simulink model "weixing3_pd_ekf1"  (R2019a)
settings: Solver=FixedStepAuto  StartTime=0.0  StopTime=40  FixedStep=0.001  RelTol=1e-3  EnableMultiTasking=on
values from neighbouring files (symbols this model uses):
  f = Jn\M(:,i)    [Copy_of_flexcont_Slidemode.m]    (also in flash.m = getframe(gcf); flexcont1_wb.m = -H'*wv(:,i); flexcont2.m; flexcont2_wb.m)
libraries: instrumentlib x2, simulink x1
settings Model: Creator=Administrator  LastModifiedBy=HP
settings DataIOCC: ExternalInput=[t, y]  LimitDataPoints=on  MaxDataPoints=15000  ReturnWorkspaceOutputs=off
settings OptimizationCC: LifeSpan=inf
settings DebuggingCC: MultiTaskCondExecSysMsg=warning  MultiTaskRateTransMsg=warning  AllowSymbolicDim=off  SFUnexpectedBacktrackingDiag=warning  SFNoUnconditionalDefaultTransitionDiag=warning  SFExecutionAtInitializationDiag=none  ArithmeticOperatorsInVariantConditions=warning
settings ModelReferenceCC: PropagateSignalLabelsOutOfModel=off
settings SFSimCC: SimUseLocalCustomCode=off
settings RTWCC: RTWUseLocalCustomCode=off
settings CodeAppCC: StateflowObjectComments=on
settings GRTTargetCC: TargetLangStandard=C89/C90 (ANSI)
settings ConfigComp: CovMetricSettings=dw  CovHtmlReporting=on  CovSaveCumulativeToWorkspaceVar=on  CovSaveSingleToWorkspaceVar=on  CovExternalEMLEnable=off

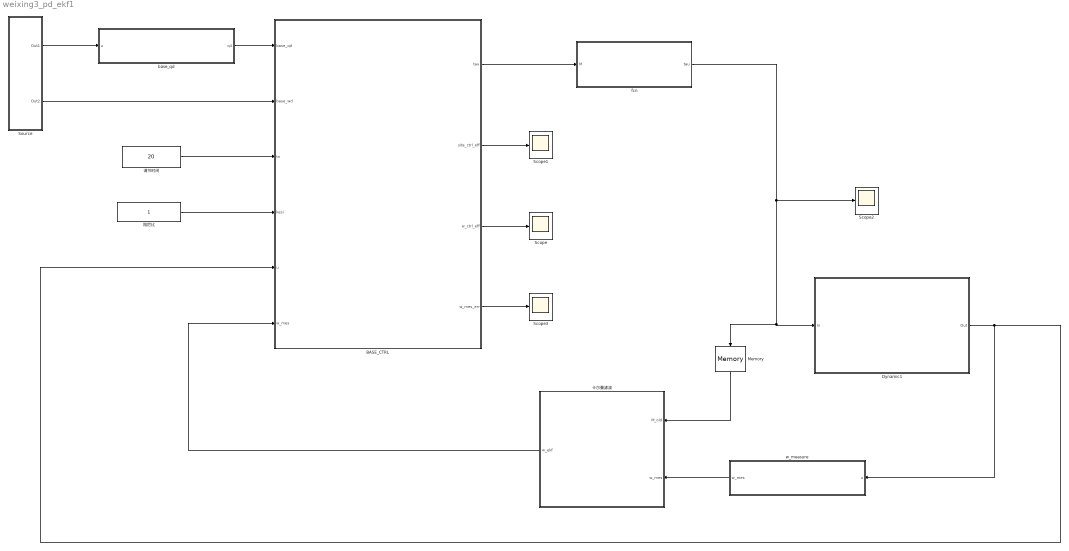
== system weixing3_pd_ekf1 ==
  " Dynamic1" : Subsystem  Description=|  mask{com_step=0.001, tcp_data_size=16, host_name=localhost, tcp_port=50028, tcp_timeout=15}
      | This block can be used to exchange data with Chrono::Engine.                                                                                      
      | A Chrono::Engine program with a running ChCosimulation inferface must be started, it will work as a server; then the Simulink program must be run.
      | Note! check that the dimensions of the exchanged vectors do match!
      mask prompts: com_step "Communication step size"; tcp_data_size "N. of scalars received from C::E (as block output)"; host_name "TCP host name (ex. 'localhost', or 'www.myhost.com')"; tcp_port "TCP port (ex. 50007)"; tcp_timeout "TCP timeout (seconds)"
      mask init:
      | block_receive = [gcb, '/TCP Receive'];
      | set_param(block_receive, 'SampleTime', num2str(com_step));
      | set_param(block_receive, 'Host', host_name);
      | set_param(block_receive, 'Port', num2str(tcp_port));
      | set_param(block_receive, 'DataSize', num2str(tcp_data_size));
      | set_param(block_receive, 'Timeout', num2str(tcp_timeout));
      | block_send = [gcb, '/TCP Send'];
      | set_param(block_send, 'Host', host_name);
      | set_param(block_send, 'Port', num2str(tcp_port));
      mask Display: disp('MBSim CoSim/Matlab')
  BASE_CTRL : MATLAB Function  TreatAsAtomicUnit=on
  Memory : Memory  InitialCondition=[zeros(9,1);1]
  Scope{,1..3} (4 alike) : Scope
  Source : Subsystem
  base_qd : MATLAB Function  TreatAsAtomicUnit=on
  fcn : MATLAB Function  TreatAsAtomicUnit=on
  w_measure : MATLAB Function  TreatAsAtomicUnit=on
  卡尔曼滤波 : MATLAB Function  TreatAsAtomicUnit=on
  调节时间 : Constant  Value=20
  阻尼比 : Constant
  wires:
  base_qd/1(q4) -> BASE_CTRL/1(base_qd)
  Source/2(Out2) -> BASE_CTRL/2(base_wd)
  调节时间/1 -> BASE_CTRL/3(tn)
  阻尼比/1 -> BASE_CTRL/4(kesi)
  BASE_CTRL/3(w_ctrl_eff) -> Scope/1
  BASE_CTRL/2(sita_ctrl_eff) -> Scope1/1
  " Dynamic1"/1(Out) -> w_measure/1(u), BASE_CTRL/5(u)
  Source/1(Out1) -> base_qd/1(u)
  BASE_CTRL/1(tau) -> fcn/1(M)
  fcn/1(tau) -> Scope2/1, Memory/1, " Dynamic1"/1(In)
  BASE_CTRL/4(w_mes_err) -> Scope3/1
  w_measure/1(w_mes) -> 卡尔曼滤波/2(w_mes)
  卡尔曼滤波/1(w_ekf) -> BASE_CTRL/6(w_mes)
  Memory/1 -> 卡尔曼滤波/1(M_old)

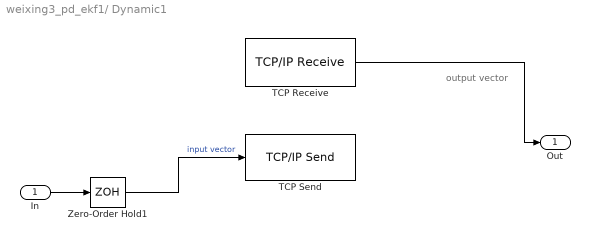
== system weixing3_pd_ekf1/ Dynamic1 ==
  note: output vector
  In : Inport
  TCP Receive : instrumentlib/TCP//IP Receive  Priority=1  Host=localhost  Port=50028  DataSize=16  EnableBlockingMode=on  Timeout=15  SampleTime=0.001  DataType=double  ByteOrder=LittleEndian  ASCIIFormatting=%f,  Terminator=LF
      settings: SourceProductName=Instrument Control Toolbox
  TCP Send : instrumentlib/TCP//IP Send  Priority=2  Host=localhost  Port=50028  EnableBlockingMode=off  Timeout=10  ByteOrder=LittleEndian  TransferDelay=on
      settings: SourceProductName=Instrument Control Toolbox
  Zero-Order Hold1 : ZeroOrderHold  SampleTime=com_step
  Out : Outport
  wires:
  Zero-Order Hold1/1 -> TCP Send/1  "input vector"
  In/1 -> Zero-Order Hold1/1
  TCP Receive/1 -> Out/1

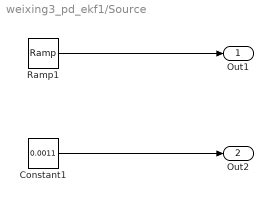
== system weixing3_pd_ekf1/Source ==
  Constant1 : Constant  Value=0.0011
  Ramp1 : simulink/Sources/Ramp  slope=0.0011  start=0  InitialOutput=0
  Out1 : Outport
  Out2 : Outport  Port=2
  wires:
  Constant1/1 -> Out2/1
  Ramp1/1 -> Out1/1

== matlab function weixing3_pd_ekf1/base_qd ==
  data: u input; q4 output
function q4 = fcn(u)
    base_qd=zeros(4,1);
    base_qd(1)=cos(u/2);
    base_qd(2)=sin(u/2);
    q1=[cos(-10*pi/180/2);0;sin(-10*pi/180/2);0];
    q2=[cos(-10*pi/180/2);sin(-10*pi/180/2);0;0];
    q3=[q1(1) -q1(2) -q1(3) -q1(4);
    q1(2) q1(1) -q1(4) q1(3);
    q1(3) q1(4) q1(1) -q1(2);
    q1(4) -q1(3) q1(2) q1(1)]*q2;
    q4=[q3(1) -q3(2) -q3(3) -q3(4);
    q3(2) q3(1) -q3(4) q3(3);
    q3(3) q3(4) q3(1) -q3(2);
    q3(4) -q3(3) q3(2) q3(1)]*base_qd;
end

== matlab function weixing3_pd_ekf1/w_measure ==
  data: u input; w_mes output
function w_mes = fcn(u)
base_q=u(6:9);
base_qv=u(13:16);
w=2*[-base_q(2),base_q(1),base_q(4),-base_q(3);
    -base_q(3),-base_q(4),base_q(1),base_q(2);
    -base_q(4),base_q(3),-base_q(2),base_q(1)]*base_qv;
noise_mes=8e-04;%1sigm  0.1deg/s(3sigm)
w_mes=w+noise_mes*randn(3,1);
end

== matlab function weixing3_pd_ekf1/BASE_CTRL ==
  data: tau output; sita_ctrl_eff output; w_ctrl_eff output; base_qd input; base_wd input; tn input; kesi input; u input; w_mes input; w_mes_err output
function [tau,sita_ctrl_eff,w_ctrl_eff,w_mes_err]  =fcn(base_qd,base_wd,tn,kesi,u,w_mes)
%%%%%MBSim输出信息
time=u(1);
time_step=u(2);
base_p=u(3:5);
base_q=u(6:9);
base_pv=u(10:12);
base_qv=u(13:16);

% %测量星体角速度（在本体系下）/滤波得到
w=w_mes;

%构造角速度叉乘矩阵
W=[0 -w(3) w(2);w(3) 0 -w(1);-w(2) w(1) 0];
%四元数误差
qe=[base_qd(1),base_qd(2),base_qd(3),base_qd(4);
    -base_qd(2),base_qd(1),base_qd(4),-base_qd(3);
    -base_qd(3),-base_qd(4),base_qd(1),base_qd(2);
    -base_qd(4),base_qd(3),-base_qd(2),base_qd(1)]*base_q;
%取矢量部分
qe1=qe(2:4);
%期望的姿态变换矩阵
A_OBd=[1-2*base_qd(3)^2-2*base_qd(4)^2,2*(base_qd(2)*base_qd(3)-base_qd(1)*base_qd(4)),2*(base_qd(2)*base_qd(4)+base_qd(1)*base_qd(3));
    2*(base_qd(2)*base_qd(3)+base_qd(1)*base_qd(4)),1-2*base_qd(2)^2-2*base_qd(4)^2,2*(base_qd(4)*base_qd(3)-base_qd(1)*base_qd(2));
    2*(base_qd(2)*base_qd(4)-base_qd(1)*base_qd(3)),2*(base_qd(4)*base_qd(3)+base_qd(1)*base_qd(2)),1-2*base_qd(2)^2-2*base_qd(3)^2];
%实际的基体姿态变换矩阵(相对于惯性坐标系)
A_OB=[1-2*base_q(3)^2-2*base_q(4)^2,2*(base_q(2)*base_q(3)-base_q(1)*base_q(4)),2*(base_q(2)*base_q(4)+base_q(1)*base_q(3));
    2*(base_q(2)*base_q(3)+base_q(1)*base_q(4)),1-2*base_q(2)^2-2*base_q(4)^2,2*(base_q(4)*base_q(3)-base_q(1)*base_q(2));
    2*(base_q(2)*base_q(4)-base_q(1)*base_q(3)),2*(base_q(4)*base_q(3)+base_q(1)*base_q(2)),1-2*base_q(2)^2-2*base_q(3)^2];
A_dB=A_OBd\A_OB;%(由误差四元数构成的姿态变换矩阵)
%角速率误差
we=w-[base_wd;0;0];

% %计算固有频率
wn=10/(kesi*tn);
%%%%%%%%%%%%%%控制率设计
%参数选取与计算
k=wn^2*2;
d=2*kesi*wn;
Jn=[566.7165 -3.77077 -3.77077;-3.77077 3658.9667 -3.77077;-3.77077 -3.77077 3705.628];
D=d*Jn;
K4=k*Jn;
%控制率
tau=zeros(3,1);
tau(1:3)=W*Jn*w-K4*qe1-D*we;

%输出指标-欧拉角误差
%根据本体和期望之间的姿态变换矩阵求解欧拉角
sita_ze=atan(-A_dB(1,2)/A_dB(1,1));
sita_ye=asin(A_dB(1,3));
sita_xe=-asin(A_dB(2,3)/cos(sita_ye));
%输出角度单位
sita_ctrl_eff=[sita_xe;sita_ye;sita_ze]*180/pi;
%输出指标-角速度
w_actual=2*[-base_q(2),base_q(1),base_q(4),-base_q(3);
    -base_q(3),-base_q(4),base_q(1),base_q(2);
    -base_q(4),base_q(3),-base_q(2),base_q(1)]*base_qv;
w_ctrl_eff=[w_actual;[base_wd;0;0]]*180/pi;
%输出指标-测量误差
w_mes_err=(w-w_actual)*180/pi;

end

== matlab function weixing3_pd_ekf1/卡尔曼滤波 ==
  data: M_old input; w_mes input; w_ekf output
function w_ekf  = fcn(M_old,w_mes)
%参数设置
noise_mes=8e-04;%1sigm
T=0.001;
%初值
persistent X;
if isempty(X)
    X=[0;0;0];
end 
persistent P;
if isempty(P)
    P=100*eye(3);
end 
%程序主体
w_old=X;
% Q=diag([1e-9,1e-9,1e-9])/1e3;
R=diag([(noise_mes)^2;(noise_mes)^2;(noise_mes)^2]);
Jn=[566.7165 -3.77077 -3.77077;-3.77077 3658.9667 -3.77077;-3.77077 -3.77077 3705.628];
JJ=inv(Jn);
W_old=[0 -w_old(3) w_old(2);w_old(3) 0 -w_old(1);-w_old(2) w_old(1) 0];
%一步预测
X=w_old-T*JJ*W_old*Jn*w_old+T*JJ*M_old(1:3);
%对非线性函数进行一阶泰勒展开
Ix=Jn(1,1);Iy=Jn(2,2);Iz=Jn(3,3);
Ixy=-Jn(1,2);Ixz=-Jn(1,3);Iyz=-Jn(2,3);
wox=w_old(1);
woy=w_old(2);
woz=w_old(3);
F=[ woy*((Iy*T*(Ixz*Iy + Ixy*Iyz))/(Iz*Ixy^2 + 2*Ixy*Ixz*Iyz + Iy*Ixz^2 + Ix*Iyz^2 - Ix*Iy*Iz) + (Iyz*T*(Ixz*Iyz + Ixy*Iz))/(Iz*Ixy^2 + 2*Ixy*Ixz*Iyz + Iy*Ixz^2 + Ix*Iyz^2 - Ix*Iy*Iz)) - wox*((Ixy*T*(Ixz*Iy + Ixy*Iyz))/(Iz*Ixy^2 + 2*Ixy*Ixz*Iyz + Iy*Ixz^2 + Ix*Iyz^2 - Ix*Iy*Iz) - (Ixz*T*(Ixz*Iyz + Ixy*Iz))/(Iz*Ixy^2 + 2*Ixy*Ixz*Iyz + Iy*Ixz^2 + Ix*Iyz^2 - Ix*Iy*Iz)) - woz*((Iyz*T*(Ixz*Iy + Ixy*Iyz))/(Iz*Ixy^2 + 2*Ixy*Ixz*Iyz + Iy*Ixz^2 + Ix*Iyz^2 - Ix*Iy*Iz) + (Iz*T*(Ixz*Iyz + Ixy*Iz))/(Iz*Ixy^2 + 2*Ixy*Ixz*Iyz + Iy*Ixz^2 + Ix*Iyz^2 - Ix*Iy*Iz)) - Ix*((T*woy*(Ixz*Iy + Ixy*Iyz))/(Iz*Ixy^2 + 2*Ixy*Ixz*Iyz + Iy*Ixz^2 + Ix*Iyz^2 - Ix*Iy*Iz) - (T*woz*(Ixz*Iyz + Ixy*Iz))/(Iz*Ixy^2 + 2*Ixy*Ixz*Iyz + Iy*Ixz^2 + Ix*Iyz^2 - Ix*Iy*Iz)) - Ixy*((T*woz*(Iyz^2 - Iy*Iz))/(Iz*Ixy^2 + 2*Ixy*Ixz*Iyz + Iy*Ixz^2 + Ix*Iyz^2 - Ix*Iy*Iz) + (T*wox*(Ixz*Iy + Ixy*Iyz))/(Iz*Ixy^2 + 2*Ixy*Ixz*Iyz + Iy*Ixz^2 + Ix*Iyz^2 - Ix*Iy*Iz)) + Ixz*((T*woy*(Iyz^2 - Iy*Iz))/(Iz*Ixy^2 + 2*Ixy*Ixz*Iyz + Iy*Ixz^2 + Ix*Iyz^2 - Ix*Iy*Iz) + (T*wox*(Ixz*Iyz + Ixy*Iz))/(Iz*Ixy^2 + 2*Ixy*Ixz*Iyz + Iy*Ixz^2 + Ix*Iyz^2 - Ix*Iy*Iz)) + 1,              Ixy*((T*woy*(Ixz*Iy + Ixy*Iyz))/(Iz*Ixy^2 + 2*Ixy*Ixz*Iyz + Iy*Ixz^2 + Ix*Iyz^2 - Ix*Iy*Iz) - (T*woz*(Ixz*Iyz + Ixy*Iz))/(Iz*Ixy^2 + 2*Ixy*Ixz*Iyz + Iy*Ixz^2 + Ix*Iyz^2 - Ix*Iy*Iz)) + wox*((Ixz*T*(Iyz^2 - Iy*Iz))/(Iz*Ixy^2 + 2*Ixy*Ixz*Iyz + Iy*Ixz^2 + Ix*Iyz^2 - Ix*Iy*Iz) - (Ix*T*(Ixz*Iy + Ixy*Iyz))/(Iz*Ixy^2 + 2*Ixy*Ixz*Iyz + Iy*Ixz^2 + Ix*Iyz^2 - Ix*Iy*Iz)) + woy*((Iyz*T*(Iyz^2 - Iy*Iz))/(Iz*Ixy^2 + 2*Ixy*Ixz*Iyz + Iy*Ixz^2 + Ix*Iyz^2 - Ix*Iy*Iz) + (Ixy*T*(Ixz*Iy + Ixy*Iyz))/(Iz*Ixy^2 + 2*Ixy*Ixz*Iyz + Iy*Ixz^2 + Ix*Iyz^2 - Ix*Iy*Iz)) - woz*((Iz*T*(Iyz^2 - Iy*Iz))/(Iz*Ixy^2 + 2*Ixy*Ixz*Iyz + Iy*Ixz^2 + Ix*Iyz^2 - Ix*Iy*Iz) - (Ixz*T*(Ixz*Iy + Ixy*Iyz))/(Iz*Ixy^2 + 2*Ixy*Ixz*Iyz + Iy*Ixz^2 + Ix*Iyz^2 - Ix*Iy*Iz)) + Iy*((T*woz*(Iyz^2 - Iy*Iz))/(Iz*Ixy^2 + 2*Ixy*Ixz*Iyz + Iy*Ixz^2 + Ix*Iyz^2 - Ix*Iy*Iz) + (T*wox*(Ixz*Iy + Ixy*Iyz))/(Iz*Ixy^2 + 2*Ixy*Ixz*Iyz + Iy*Ixz^2 + Ix*Iyz^2 - Ix*Iy*Iz)) + Iyz*((T*woy*(Iyz^2 - Iy*Iz))/(Iz*Ixy^2 + 2*Ixy*Ixz*Iyz + Iy*Ixz^2 + Ix*Iyz^2 - Ix*Iy*Iz) + (T*wox*(Ixz*Iyz + Ixy*Iz))/(Iz*Ixy^2 + 2*Ixy*Ixz*Iyz + Iy*Ixz^2 + Ix*Iyz^2 - Ix*Iy*Iz)),              Ixz*((T*woy*(Ixz*Iy + Ixy*Iyz))/(Iz*Ixy^2 + 2*Ixy*Ixz*Iyz + Iy*Ixz^2 + Ix*Iyz^2 - Ix*Iy*Iz) - (T*woz*(Ixz*Iyz + Ixy*Iz))/(Iz*Ixy^2 + 2*Ixy*Ixz*Iyz + Iy*Ixz^2 + Ix*Iyz^2 - Ix*Iy*Iz)) - wox*((Ixy*T*(Iyz^2 - Iy*Iz))/(Iz*Ixy^2 + 2*Ixy*Ixz*Iyz + Iy*Ixz^2 + Ix*Iyz^2 - Ix*Iy*Iz) - (Ix*T*(Ixz*Iyz + Ixy*Iz))/(Iz*Ixy^2 + 2*Ixy*Ixz*Iyz + Iy*Ixz^2 + Ix*Iyz^2 - Ix*Iy*Iz)) + woy*((Iy*T*(Iyz^2 - Iy*Iz))/(Iz*Ixy^2 + 2*Ixy*Ixz*Iyz + Iy*Ixz^2 + Ix*Iyz^2 - Ix*Iy*Iz) - (Ixy*T*(Ixz*Iyz + Ixy*Iz))/(Iz*Ixy^2 + 2*Ixy*Ixz*Iyz + Iy*Ixz^2 + Ix*Iyz^2 - Ix*Iy*Iz)) - woz*((Iyz*T*(Iyz^2 - Iy*Iz))/(Iz*Ixy^2 + 2*Ixy*Ixz*Iyz + Iy*Ixz^2 + Ix*Iyz^2 - Ix*Iy*Iz) + (Ixz*T*(Ixz*Iyz + Ixy*Iz))/(Iz*Ixy^2 + 2*Ixy*Ixz*Iyz + Iy*Ixz^2 + Ix*Iyz^2 - Ix*Iy*Iz)) - Iyz*((T*woz*(Iyz^2 - Iy*Iz))/(Iz*Ixy^2 + 2*Ixy*Ixz*Iyz + Iy*Ixz^2 + Ix*Iyz^2 - Ix*Iy*Iz) + (T*wox*(Ixz*Iy + Ixy*Iyz))/(Iz*Ixy^2 + 2*Ixy*Ixz*Iyz + Iy*Ixz^2 + Ix*Iyz^2 - Ix*Iy*Iz)) - Iz*((T*woy*(Iyz^2 - Iy*Iz))/(Iz*Ixy^2 + 2*Ixy*Ixz*Iyz + Iy*Ixz^2 + Ix*Iyz^2 - Ix*Iy*Iz) + (T*wox*(Ixz*Iyz + Ixy*Iz))/(Iz*Ixy^2 + 2*Ixy*Ixz*Iyz + Iy*Ixz^2 + Ix*Iyz^2 - Ix*Iy*Iz));
              woz*((Iz*T*(Ixz^2 - Ix*Iz))/(Iz*Ixy^2 + 2*Ixy*Ixz*Iyz + Iy*Ixz^2 + Ix*Iyz^2 - Ix*Iy*Iz) - (Iyz*T*(Ixy*Ixz + Ix*Iyz))/(Iz*Ixy^2 + 2*Ixy*Ixz*Iyz + Iy*Ixz^2 + Ix*Iyz^2 - Ix*Iy*Iz)) - wox*((Ixz*T*(Ixz^2 - Ix*Iz))/(Iz*Ixy^2 + 2*Ixy*Ixz*Iyz + Iy*Ixz^2 + Ix*Iyz^2 - Ix*Iy*Iz) + (Ixy*T*(Ixy*Ixz + Ix*Iyz))/(Iz*Ixy^2 + 2*Ixy*Ixz*Iyz + Iy*Ixz^2 + Ix*Iyz^2 - Ix*Iy*Iz)) - woy*((Iyz*T*(Ixz^2 - Ix*Iz))/(Iz*Ixy^2 + 2*Ixy*Ixz*Iyz + Iy*Ixz^2 + Ix*Iyz^2 - Ix*Iy*Iz) - (Iy*T*(Ixy*Ixz + Ix*Iyz))/(Iz*Ixy^2 + 2*Ixy*Ixz*Iyz + Iy*Ixz^2 + Ix*Iyz^2 - Ix*Iy*Iz)) - Ixy*((T*wox*(Ixy*Ixz + Ix*Iyz))/(Iz*Ixy^2 + 2*Ixy*Ixz*Iyz + Iy*Ixz^2 + Ix*Iyz^2 - Ix*Iy*Iz) - (T*woz*(Ixz*Iyz + Ixy*Iz))/(Iz*Ixy^2 + 2*Ixy*Ixz*Iyz + Iy*Ixz^2 + Ix*Iyz^2 - Ix*Iy*Iz)) - Ix*((T*woz*(Ixz^2 - Ix*Iz))/(Iz*Ixy^2 + 2*Ixy*Ixz*Iyz + Iy*Ixz^2 + Ix*Iyz^2 - Ix*Iy*Iz) + (T*woy*(Ixy*Ixz + Ix*Iyz))/(Iz*Ixy^2 + 2*Ixy*Ixz*Iyz + Iy*Ixz^2 + Ix*Iyz^2 - Ix*Iy*Iz)) - Ixz*((T*wox*(Ixz^2 - Ix*Iz))/(Iz*Ixy^2 + 2*Ixy*Ixz*Iyz + Iy*Ixz^2 + Ix*Iyz^2 - Ix*Iy*Iz) + (T*woy*(Ixz*Iyz + Ixy*Iz))/(Iz*Ixy^2 + 2*Ixy*Ixz*Iyz + Iy*Ixz^2 + Ix*Iyz^2 - Ix*Iy*Iz)), woy*((Ixy*T*(Ixy*Ixz + Ix*Iyz))/(Iz*Ixy^2 + 2*Ixy*Ixz*Iyz + Iy*Ixz^2 + Ix*Iyz^2 - Ix*Iy*Iz) - (Iyz*T*(Ixz*Iyz + Ixy*Iz))/(Iz*Ixy^2 + 2*Ixy*Ixz*Iyz + Iy*Ixz^2 + Ix*Iyz^2 - Ix*Iy*Iz)) - wox*((Ix*T*(Ixy*Ixz + Ix*Iyz))/(Iz*Ixy^2 + 2*Ixy*Ixz*Iyz + Iy*Ixz^2 + Ix*Iyz^2 - Ix*Iy*Iz) + (Ixz*T*(Ixz*Iyz + Ixy*Iz))/(Iz*Ixy^2 + 2*Ixy*Ixz*Iyz + Iy*Ixz^2 + Ix*Iyz^2 - Ix*Iy*Iz)) + woz*((Ixz*T*(Ixy*Ixz + Ix*Iyz))/(Iz*Ixy^2 + 2*Ixy*Ixz*Iyz + Iy*Ixz^2 + Ix*Iyz^2 - Ix*Iy*Iz) + (Iz*T*(Ixz*Iyz + Ixy*Iz))/(Iz*Ixy^2 + 2*Ixy*Ixz*Iyz + Iy*Ixz^2 + Ix*Iyz^2 - Ix*Iy*Iz)) + Iy*((T*wox*(Ixy*Ixz + Ix*Iyz))/(Iz*Ixy^2 + 2*Ixy*Ixz*Iyz + Iy*Ixz^2 + Ix*Iyz^2 - Ix*Iy*Iz) - (T*woz*(Ixz*Iyz + Ixy*Iz))/(Iz*Ixy^2 + 2*Ixy*Ixz*Iyz + Iy*Ixz^2 + Ix*Iyz^2 - Ix*Iy*Iz)) + Ixy*((T*woz*(Ixz^2 - Ix*Iz))/(Iz*Ixy^2 + 2*Ixy*Ixz*Iyz + Iy*Ixz^2 + Ix*Iyz^2 - Ix*Iy*Iz) + (T*woy*(Ixy*Ixz + Ix*Iyz))/(Iz*Ixy^2 + 2*Ixy*Ixz*Iyz + Iy*Ixz^2 + Ix*Iyz^2 - Ix*Iy*Iz)) - Iyz*((T*wox*(Ixz^2 - Ix*Iz))/(Iz*Ixy^2 + 2*Ixy*Ixz*Iyz + Iy*Ixz^2 + Ix*Iyz^2 - Ix*Iy*Iz) + (T*woy*(Ixz*Iyz + Ixy*Iz))/(Iz*Ixy^2 + 2*Ixy*Ixz*Iyz + Iy*Ixz^2 + Ix*Iyz^2 - Ix*Iy*Iz)) + 1,              woy*((Ixy*T*(Ixz^2 - Ix*Iz))/(Iz*Ixy^2 + 2*Ixy*Ixz*Iyz + Iy*Ixz^2 + Ix*Iyz^2 - Ix*Iy*Iz) - (Iy*T*(Ixz*Iyz + Ixy*Iz))/(Iz*Ixy^2 + 2*Ixy*Ixz*Iyz + Iy*Ixz^2 + Ix*Iyz^2 - Ix*Iy*Iz)) - wox*((Ix*T*(Ixz^2 - Ix*Iz))/(Iz*Ixy^2 + 2*Ixy*Ixz*Iyz + Iy*Ixz^2 + Ix*Iyz^2 - Ix*Iy*Iz) - (Ixy*T*(Ixz*Iyz + Ixy*Iz))/(Iz*Ixy^2 + 2*Ixy*Ixz*Iyz + Iy*Ixz^2 + Ix*Iyz^2 - Ix*Iy*Iz)) - Iyz*((T*wox*(Ixy*Ixz + Ix*Iyz))/(Iz*Ixy^2 + 2*Ixy*Ixz*Iyz + Iy*Ixz^2 + Ix*Iyz^2 - Ix*Iy*Iz) - (T*woz*(Ixz*Iyz + Ixy*Iz))/(Iz*Ixy^2 + 2*Ixy*Ixz*Iyz + Iy*Ixz^2 + Ix*Iyz^2 - Ix*Iy*Iz)) + woz*((Ixz*T*(Ixz^2 - Ix*Iz))/(Iz*Ixy^2 + 2*Ixy*Ixz*Iyz + Iy*Ixz^2 + Ix*Iyz^2 - Ix*Iy*Iz) + (Iyz*T*(Ixz*Iyz + Ixy*Iz))/(Iz*Ixy^2 + 2*Ixy*Ixz*Iyz + Iy*Ixz^2 + Ix*Iyz^2 - Ix*Iy*Iz)) + Ixz*((T*woz*(Ixz^2 - Ix*Iz))/(Iz*Ixy^2 + 2*Ixy*Ixz*Iyz + Iy*Ixz^2 + Ix*Iyz^2 - Ix*Iy*Iz) + (T*woy*(Ixy*Ixz + Ix*Iyz))/(Iz*Ixy^2 + 2*Ixy*Ixz*Iyz + Iy*Ixz^2 + Ix*Iyz^2 - Ix*Iy*Iz)) + Iz*((T*wox*(Ixz^2 - Ix*Iz))/(Iz*Ixy^2 + 2*Ixy*Ixz*Iyz + Iy*Ixz^2 + Ix*Iyz^2 - Ix*Iy*Iz) + (T*woy*(Ixz*Iyz + Ixy*Iz))/(Iz*Ixy^2 + 2*Ixy*Ixz*Iyz + Iy*Ixz^2 + Ix*Iyz^2 - Ix*Iy*Iz));
             Ixz*((T*wox*(Ixy*Ixz + Ix*Iyz))/(Iz*Ixy^2 + 2*Ixy*Ixz*Iyz + Iy*Ixz^2 + Ix*Iyz^2 - Ix*Iy*Iz) - (T*woy*(Ixz*Iy + Ixy*Iyz))/(Iz*Ixy^2 + 2*Ixy*Ixz*Iyz + Iy*Ixz^2 + Ix*Iyz^2 - Ix*Iy*Iz)) + wox*((Ixy*T*(Ixy^2 - Ix*Iy))/(Iz*Ixy^2 + 2*Ixy*Ixz*Iyz + Iy*Ixz^2 + Ix*Iyz^2 - Ix*Iy*Iz) + (Ixz*T*(Ixy*Ixz + Ix*Iyz))/(Iz*Ixy^2 + 2*Ixy*Ixz*Iyz + Iy*Ixz^2 + Ix*Iyz^2 - Ix*Iy*Iz)) - woy*((Iy*T*(Ixy^2 - Ix*Iy))/(Iz*Ixy^2 + 2*Ixy*Ixz*Iyz + Iy*Ixz^2 + Ix*Iyz^2 - Ix*Iy*Iz) - (Iyz*T*(Ixy*Ixz + Ix*Iyz))/(Iz*Ixy^2 + 2*Ixy*Ixz*Iyz + Iy*Ixz^2 + Ix*Iyz^2 - Ix*Iy*Iz)) + woz*((Iyz*T*(Ixy^2 - Ix*Iy))/(Iz*Ixy^2 + 2*Ixy*Ixz*Iyz + Iy*Ixz^2 + Ix*Iyz^2 - Ix*Iy*Iz) - (Iz*T*(Ixy*Ixz + Ix*Iyz))/(Iz*Ixy^2 + 2*Ixy*Ixz*Iyz + Iy*Ixz^2 + Ix*Iyz^2 - Ix*Iy*Iz)) + Ix*((T*woy*(Ixy^2 - Ix*Iy))/(Iz*Ixy^2 + 2*Ixy*Ixz*Iyz + Iy*Ixz^2 + Ix*Iyz^2 - Ix*Iy*Iz) + (T*woz*(Ixy*Ixz + Ix*Iyz))/(Iz*Ixy^2 + 2*Ixy*Ixz*Iyz + Iy*Ixz^2 + Ix*Iyz^2 - Ix*Iy*Iz)) + Ixy*((T*wox*(Ixy^2 - Ix*Iy))/(Iz*Ixy^2 + 2*Ixy*Ixz*Iyz + Iy*Ixz^2 + Ix*Iyz^2 - Ix*Iy*Iz) + (T*woz*(Ixz*Iy + Ixy*Iyz))/(Iz*Ixy^2 + 2*Ixy*Ixz*Iyz + Iy*Ixz^2 + Ix*Iyz^2 - Ix*Iy*Iz)),              Iyz*((T*wox*(Ixy*Ixz + Ix*Iyz))/(Iz*Ixy^2 + 2*Ixy*Ixz*Iyz + Iy*Ixz^2 + Ix*Iyz^2 - Ix*Iy*Iz) - (T*woy*(Ixz*Iy + Ixy*Iyz))/(Iz*Ixy^2 + 2*Ixy*Ixz*Iyz + Iy*Ixz^2 + Ix*Iyz^2 - Ix*Iy*Iz)) + wox*((Ix*T*(Ixy^2 - Ix*Iy))/(Iz*Ixy^2 + 2*Ixy*Ixz*Iyz + Iy*Ixz^2 + Ix*Iyz^2 - Ix*Iy*Iz) - (Ixz*T*(Ixz*Iy + Ixy*Iyz))/(Iz*Ixy^2 + 2*Ixy*Ixz*Iyz + Iy*Ixz^2 + Ix*Iyz^2 - Ix*Iy*Iz)) - woy*((Ixy*T*(Ixy^2 - Ix*Iy))/(Iz*Ixy^2 + 2*Ixy*Ixz*Iyz + Iy*Ixz^2 + Ix*Iyz^2 - Ix*Iy*Iz) + (Iyz*T*(Ixz*Iy + Ixy*Iyz))/(Iz*Ixy^2 + 2*Ixy*Ixz*Iyz + Iy*Ixz^2 + Ix*Iyz^2 - Ix*Iy*Iz)) - woz*((Ixz*T*(Ixy^2 - Ix*Iy))/(Iz*Ixy^2 + 2*Ixy*Ixz*Iyz + Iy*Ixz^2 + Ix*Iyz^2 - Ix*Iy*Iz) - (Iz*T*(Ixz*Iy + Ixy*Iyz))/(Iz*Ixy^2 + 2*Ixy*Ixz*Iyz + Iy*Ixz^2 + Ix*Iyz^2 - Ix*Iy*Iz)) - Ixy*((T*woy*(Ixy^2 - Ix*Iy))/(Iz*Ixy^2 + 2*Ixy*Ixz*Iyz + Iy*Ixz^2 + Ix*Iyz^2 - Ix*Iy*Iz) + (T*woz*(Ixy*Ixz + Ix*Iyz))/(Iz*Ixy^2 + 2*Ixy*Ixz*Iyz + Iy*Ixz^2 + Ix*Iyz^2 - Ix*Iy*Iz)) - Iy*((T*wox*(Ixy^2 - Ix*Iy))/(Iz*Ixy^2 + 2*Ixy*Ixz*Iyz + Iy*Ixz^2 + Ix*Iyz^2 - Ix*Iy*Iz) + (T*woz*(Ixz*Iy + Ixy*Iyz))/(Iz*Ixy^2 + 2*Ixy*Ixz*Iyz + Iy*Ixz^2 + Ix*Iyz^2 - Ix*Iy*Iz)), wox*((Ix*T*(Ixy*Ixz + Ix*Iyz))/(Iz*Ixy^2 + 2*Ixy*Ixz*Iyz + Iy*Ixz^2 + Ix*Iyz^2 - Ix*Iy*Iz) + (Ixy*T*(Ixz*Iy + Ixy*Iyz))/(Iz*Ixy^2 + 2*Ixy*Ixz*Iyz + Iy*Ixz^2 + Ix*Iyz^2 - Ix*Iy*Iz)) - woy*((Ixy*T*(Ixy*Ixz + Ix*Iyz))/(Iz*Ixy^2 + 2*Ixy*Ixz*Iyz + Iy*Ixz^2 + Ix*Iyz^2 - Ix*Iy*Iz) + (Iy*T*(Ixz*Iy + Ixy*Iyz))/(Iz*Ixy^2 + 2*Ixy*Ixz*Iyz + Iy*Ixz^2 + Ix*Iyz^2 - Ix*Iy*Iz)) - woz*((Ixz*T*(Ixy*Ixz + Ix*Iyz))/(Iz*Ixy^2 + 2*Ixy*Ixz*Iyz + Iy*Ixz^2 + Ix*Iyz^2 - Ix*Iy*Iz) - (Iyz*T*(Ixz*Iy + Ixy*Iyz))/(Iz*Ixy^2 + 2*Ixy*Ixz*Iyz + Iy*Ixz^2 + Ix*Iyz^2 - Ix*Iy*Iz)) - Iz*((T*wox*(Ixy*Ixz + Ix*Iyz))/(Iz*Ixy^2 + 2*Ixy*Ixz*Iyz + Iy*Ixz^2 + Ix*Iyz^2 - Ix*Iy*Iz) - (T*woy*(Ixz*Iy + Ixy*Iyz))/(Iz*Ixy^2 + 2*Ixy*Ixz*Iyz + Iy*Ixz^2 + Ix*Iyz^2 - Ix*Iy*Iz)) - Ixz*((T*woy*(Ixy^2 - Ix*Iy))/(Iz*Ixy^2 + 2*Ixy*Ixz*Iyz + Iy*Ixz^2 + Ix*Iyz^2 - Ix*Iy*Iz) + (T*woz*(Ixy*Ixz + Ix*Iyz))/(Iz*Ixy^2 + 2*Ixy*Ixz*Iyz + Iy*Ixz^2 + Ix*Iyz^2 - Ix*Iy*Iz)) + Iyz*((T*wox*(Ixy^2 - Ix*Iy))/(Iz*Ixy^2 + 2*Ixy*Ixz*Iyz + Iy*Ixz^2 + Ix*Iyz^2 - Ix*Iy*Iz) + (T*woz*(Ixz*Iy + Ixy*Iyz))/(Iz*Ixy^2 + 2*Ixy*Ixz*Iyz + Iy*Ixz^2 + Ix*Iyz^2 - Ix*Iy*Iz)) + 1];
P=F*P*F';
h=eye(3);
K=P*h'*inv(h*P*h'+R);
X=X+K*(w_mes-h*X);
P=(eye(3)-K*h)*P;
w_ekf=X;
end

== matlab function weixing3_pd_ekf1/fcn ==
  data: M input; tau output
function tau = fcn(M)


tau=[M(1);M(2);M(3);zeros(6,1);1];
end
